simulink model "Controller_20231019"  (R2021b)
settings: Solver=ode4  StartTime=0.0  StopTime=5  FixedStep=0.01  RelTol=1e-3
values from neighbouring files (symbols this model uses):
  diag_M = diagonalize(M_frak0, M_frak)    [Initiate_KUKA_inv.m]
  iota0 = eye(6,6)    [Initiate_KUKA_inv.m]
  K_d = 10*[1.3*eye(3) zeros(3);zeros(3) 0.8*eye(3)]    [Initiate_FQ.m]    (also in Initiate_KUKA_inv.m = 5*[0.7*eye(3) zeros(3);zeros(3) 0.5*eye(3)])
  K_i = 5*[0.1*eye(3) zeros(3);zeros(3) 0.01*eye(3)]    [Initiate_FQ.m]    (also in Initiate_KUKA_inv.m = 5*[0.01*eye(3) zeros(3);zeros(3) 0.001*eye(3)])
  K_p = 100*[0.1 0 0 0 0 0;0 0.1 0 0 0 0; 0 0 0.1 0 0 0; 0 0 0 0.01 0 0 ... (first row only)    [Initiate_FQ.m]    (also in Initiate_KUKA_inv.m = 5*[0.1 0 0 0 0 0;0 0.1 0 0 0 0; 0 0 0.1 0 0 0; 0 0 0 0.01 0 )
  m0 = robot.Bodies{1,n+1}.Mass    [Initiate_KUKA_inv.m]
  M_t = (((Adjoint(g_It))'\M_t_body)/(Adjoint(g_It)))    [Initiate_FQ.m]    (also in Initiate_KUKA_inv.m = [eye(3)*mt zeros(3); zeros(3) eye(3)*80])
  mm = zeros(1,n)    [Initiate_KUKA_inv.m]
  mu = P0    [Initiate_FQ.m]    (also in Initiate_KUKA_inv.m = zeros(6,1))
  mu_t = inv((Adjoint(g_It))')*M_t_body*[V_It;w_t]    [Initiate_FQ.m]    (also in Initiate_KUKA_inv.m = M_t*[V_0t;w_t])
  q_dot_m = [0;0;0;0;0;0;0]    [Initiate_FQ.m]    (also in Initiate_KUKA_inv.m)
  q_m = [0.2;1.2;0.3;2.5;0.5;1.5;0.6]    [Initiate_FQ.m]    (also in Initiate_KUKA_inv.m = [0;0;0;0;0;0;0])
  rho_0t = [0.24;0.26;0.25]    [Initiate_KUKA_inv.m]
  sc_size = 1    [Initiate_KUKA_inv.m]
  V_0t = [-0.01;-0.01;0]    [Initiate_KUKA_inv.m]
  V_I0 = [-0.001;-0.001;0.0;-0.001;0.001;0.002]    [Initiate_FQ.m]    (also in Initiate_KUKA_inv.m = [0;0;0;0;0;0])
  Xi_m_matrix = zeros(6*n,n)    [Initiate_KUKA_inv.m]
undefined symbols (not defined in the file or in its folder): I0, Ie, Im, me, X, Xi_m, Y, Z
libraries: nesl_utility x83, sm_lib x78, robotcorelib x4
(part 4 of 4)

== system Controller_20231019/Space Manipulator1/joint//link5/iiwa_link_5 ==
  Inertia : sm_lib/Body Elements/Inertia  InertiaType=Custom  Mass=2.1633  MassUnits=kg  CenterOfMass=[0, 0, 0]  CenterOfMassUnits=m  MomentsOfInertia=[Im(1,1,5) Im(2,2,5) Im(3,3,5)]  MomentsOfInertiaUnits=kg*m^2  ProductsOfInertia=[Im(3,2,5) Im(3,1,5) Im(2,1,5)]  ProductsOfInertiaUnits=kg*m^2  GraphicType=None  MarkerShape=Inertia  MarkerSize=20  GraphicVisPropType=SimpleVisualProperties  GraphicDiffuseColor=[0.5 0.5 0.5]  GraphicSpecularColor=[0.5 0.5 0.5 1.0]  GraphicAmbientColor=[0.15 0.15 0.15 1.0]  GraphicEmissiveColor=[0.0 0.0 0.0 1.0]  GraphicShininess=75  GraphicOpacity=1.0
  ReferenceFrame : sm_lib/Frames and Transforms/Reference Frame
  Visual : sm_lib/Body Elements/File Solid  ExtGeomFileName=iiwa_description/meshes/iiwa7/visual/link_5.stl  UnitType=Custom  ExtGeomFileUnits=m  StepReaderType=HEX  ExportConvexHullGeometry=off  InertiaType=Custom  Mass=0  MassUnits=kg  CenterOfMass=[0, 0, 0]  CenterOfMassUnits=m  MomentsOfInertia=[0, 0, 0]  MomentsOfInertiaUnits=kg*m^2  ProductsOfInertia=[0, 0, 0]  ProductsOfInertiaUnits=kg*m^2  BasedOnType=DensityFromFile  Density=1000  DensityUnits=kg/m^3  DoExposeReferenceFrame=on  SerializedFrames=<Frames/>  GraphicType=FromGeometry  MarkerShape=Sphere  MarkerSize=10  GraphicVisPropType=SimpleVisualProperties  GraphicDiffuseColor=[1, 0.423529411765, 0.0392156862745]  GraphicSpecularColor=[0.5 0.5 0.5 1.0]  GraphicAmbientColor=[0.15 0.15 0.15 1.0]  GraphicEmissiveColor=[0.0 0.0 0.0 1.0]  GraphicShininess=75  GraphicOpacity=1
  VisualOriginTransform : sm_lib/Frames and Transforms/Rigid Transform  TranslationMethod=Cartesian  TranslationStandardOffset=0  TranslationLengthUnit=m  TranslationStandardAxis=+Z  TranslationCartesianOffset=[0, 0, -0.026]  TranslationROffset=0  TranslationROffsetUnits=m  TranslationZOffset=0  TranslationZOffsetUnits=m  TranslationThetaOffset=0  TranslationThetaOffsetUnits=deg  RotationMethod=RotationSequence  RotationAngleUnits=deg  RotationStandardAxis=+Z  RotationAngle=0.0  RotationArbitraryAxis=[0 0 1]  FollAlignAxisA=+X  BaseAlignAxisA=+Y  FollAlignAxisB=+Y  BaseAlignAxisB=+Z  RotationSequenceAxes=BaseAxes  RotationSequence=XYZ  RotationSequenceAngles=[0, 0, 0]  RotationSequenceAnglesUnits=rad  RotationMatrix=[1 0 0; 0 1 0; 0 0 1]
  iiwa_joint_5_AxisInvTransform : sm_lib/Frames and Transforms/Rigid Transform  TranslationMethod=Cartesian  TranslationStandardOffset=0  TranslationLengthUnit=m  TranslationStandardAxis=+Z  TranslationCartesianOffset=[0, 0, 0]  TranslationROffset=0  TranslationROffsetUnits=m  TranslationZOffset=0  TranslationZOffsetUnits=m  TranslationThetaOffset=0  TranslationThetaOffsetUnits=deg  RotationMethod=ArbitraryAxis  RotationAngleUnits=rad  RotationStandardAxis=+Z  RotationAngle=0  RotationArbitraryAxis=[1, 0, 0]  FollAlignAxisA=+X  BaseAlignAxisA=+Y  FollAlignAxisB=+Y  BaseAlignAxisB=+Z  RotationSequenceAxes=FollowerAxes  RotationSequence=XYX  RotationSequenceAngles=[0 0 0]  RotationSequenceAnglesUnits=deg  RotationMatrix=[1 0 0; 0 1 0; 0 0 1]
  iiwa_joint_6_AxisTransform : sm_lib/Frames and Transforms/Rigid Transform  TranslationMethod=Cartesian  TranslationStandardOffset=0  TranslationLengthUnit=m  TranslationStandardAxis=+Z  TranslationCartesianOffset=[0, 0, 0]  TranslationROffset=0  TranslationROffsetUnits=m  TranslationZOffset=0  TranslationZOffsetUnits=m  TranslationThetaOffset=0  TranslationThetaOffsetUnits=deg  RotationMethod=ArbitraryAxis  RotationAngleUnits=rad  RotationStandardAxis=+Z  RotationAngle=0  RotationArbitraryAxis=[1, 0, 0]  FollAlignAxisA=+X  BaseAlignAxisA=+Y  FollAlignAxisB=+Y  BaseAlignAxisB=+Z  RotationSequenceAxes=FollowerAxes  RotationSequence=XYX  RotationSequenceAngles=[0 0 0]  RotationSequenceAnglesUnits=deg  RotationMatrix=[1 0 0; 0 1 0; 0 0 1]
  iiwa_joint_6_OriginTransform : sm_lib/Frames and Transforms/Rigid Transform  TranslationMethod=Cartesian  TranslationStandardOffset=0  TranslationLengthUnit=m  TranslationStandardAxis=+Z  TranslationCartesianOffset=[0, 0.0607 , 0.19]  TranslationROffset=0  TranslationROffsetUnits=m  TranslationZOffset=0  TranslationZOffsetUnits=m  TranslationThetaOffset=0  TranslationThetaOffsetUnits=deg  RotationMethod=RotationSequence  RotationAngleUnits=deg  RotationStandardAxis=+Z  RotationAngle=0.0  RotationArbitraryAxis=[0 0 1]  FollAlignAxisA=+X  BaseAlignAxisA=+Y  FollAlignAxisB=+Y  BaseAlignAxisB=+Z  RotationSequenceAxes=BaseAxes  RotationSequence=XYZ  RotationSequenceAngles=[1.57079632679, 0, 0]  RotationSequenceAnglesUnits=rad  RotationMatrix=[1 0 0; 0 1 0; 0 0 1]
  F : PMIOPort  Side=Left
  F1 : PMIOPort  Port=2  Side=Right
  connections:
  iiwa_joint_5_AxisInvTransform/LConn1 -- iiwa_joint_6_OriginTransform/LConn1 -- Inertia/RConn1 -- ReferenceFrame/RConn1 -- VisualOriginTransform/LConn1
  Visual/RConn1 -- VisualOriginTransform/RConn1
  iiwa_joint_5_AxisInvTransform/RConn1 -- F/RConn1
  iiwa_joint_6_AxisTransform/RConn1 -- F1/RConn1
  iiwa_joint_6_AxisTransform/LConn1 -- iiwa_joint_6_OriginTransform/RConn1

== system Controller_20231019/Space Manipulator1/joint//link6/iiwa_link_6 ==
  Inertia : sm_lib/Body Elements/Inertia  InertiaType=Custom  Mass=2.3466  MassUnits=kg  CenterOfMass=[0, 0, 0]  CenterOfMassUnits=m  MomentsOfInertia=[Im(1,1,6) Im(2,2,6) Im(3,3,6)]  MomentsOfInertiaUnits=kg*m^2  ProductsOfInertia=[Im(3,2,6) Im(3,1,6) Im(2,1,6)]  ProductsOfInertiaUnits=kg*m^2  GraphicType=None  MarkerShape=Inertia  MarkerSize=20  GraphicVisPropType=SimpleVisualProperties  GraphicDiffuseColor=[0.5 0.5 0.5]  GraphicSpecularColor=[0.5 0.5 0.5 1.0]  GraphicAmbientColor=[0.15 0.15 0.15 1.0]  GraphicEmissiveColor=[0.0 0.0 0.0 1.0]  GraphicShininess=75  GraphicOpacity=1.0
  ReferenceFrame : sm_lib/Frames and Transforms/Reference Frame
  Visual : sm_lib/Body Elements/File Solid  ExtGeomFileName=iiwa_description/meshes/iiwa7/visual/link_6.stl  UnitType=Custom  ExtGeomFileUnits=m  StepReaderType=HEX  ExportConvexHullGeometry=off  InertiaType=Custom  Mass=0  MassUnits=kg  CenterOfMass=[0, 0, 0]  CenterOfMassUnits=m  MomentsOfInertia=[0, 0, 0]  MomentsOfInertiaUnits=kg*m^2  ProductsOfInertia=[0, 0, 0]  ProductsOfInertiaUnits=kg*m^2  BasedOnType=DensityFromFile  Density=1000  DensityUnits=kg/m^3  DoExposeReferenceFrame=on  SerializedFrames=<Frames/>  GraphicType=FromGeometry  MarkerShape=Sphere  MarkerSize=10  GraphicVisPropType=SimpleVisualProperties  GraphicDiffuseColor=[1, 0.423529411765, 0.0392156862745]  GraphicSpecularColor=[0.5 0.5 0.5 1.0]  GraphicAmbientColor=[0.15 0.15 0.15 1.0]  GraphicEmissiveColor=[0.0 0.0 0.0 1.0]  GraphicShininess=75  GraphicOpacity=1
  VisualOriginTransform : sm_lib/Frames and Transforms/Rigid Transform  TranslationMethod=Cartesian  TranslationStandardOffset=0  TranslationLengthUnit=m  TranslationStandardAxis=+Z  TranslationCartesianOffset=[0, 0, 0.0607 ]  TranslationROffset=0  TranslationROffsetUnits=m  TranslationZOffset=0  TranslationZOffsetUnits=m  TranslationThetaOffset=0  TranslationThetaOffsetUnits=deg  RotationMethod=RotationSequence  RotationAngleUnits=deg  RotationStandardAxis=+Z  RotationAngle=0.0  RotationArbitraryAxis=[0 0 1]  FollAlignAxisA=+X  BaseAlignAxisA=+Y  FollAlignAxisB=+Y  BaseAlignAxisB=+Z  RotationSequenceAxes=BaseAxes  RotationSequence=XYZ  RotationSequenceAngles=[0, 0, 0]  RotationSequenceAnglesUnits=rad  RotationMatrix=[1 0 0; 0 1 0; 0 0 1]
  iiwa_joint_6_AxisInvTransform : sm_lib/Frames and Transforms/Rigid Transform  TranslationMethod=Cartesian  TranslationStandardOffset=0  TranslationLengthUnit=m  TranslationStandardAxis=+Z  TranslationCartesianOffset=[0, 0, 0]  TranslationROffset=0  TranslationROffsetUnits=m  TranslationZOffset=0  TranslationZOffsetUnits=m  TranslationThetaOffset=0  TranslationThetaOffsetUnits=deg  RotationMethod=ArbitraryAxis  RotationAngleUnits=rad  RotationStandardAxis=+Z  RotationAngle=0  RotationArbitraryAxis=[1, 0, 0]  FollAlignAxisA=+X  BaseAlignAxisA=+Y  FollAlignAxisB=+Y  BaseAlignAxisB=+Z  RotationSequenceAxes=FollowerAxes  RotationSequence=XYX  RotationSequenceAngles=[0 0 0]  RotationSequenceAnglesUnits=deg  RotationMatrix=[1 0 0; 0 1 0; 0 0 1]
  iiwa_joint_7_AxisTransform : sm_lib/Frames and Transforms/Rigid Transform  TranslationMethod=Cartesian  TranslationStandardOffset=0  TranslationLengthUnit=m  TranslationStandardAxis=+Z  TranslationCartesianOffset=[0, 0, 0]  TranslationROffset=0  TranslationROffsetUnits=m  TranslationZOffset=0  TranslationZOffsetUnits=m  TranslationThetaOffset=0  TranslationThetaOffsetUnits=deg  RotationMethod=ArbitraryAxis  RotationAngleUnits=rad  RotationStandardAxis=+Z  RotationAngle=0  RotationArbitraryAxis=[1, 0, 0]  FollAlignAxisA=+X  BaseAlignAxisA=+Y  FollAlignAxisB=+Y  BaseAlignAxisB=+Z  RotationSequenceAxes=FollowerAxes  RotationSequence=XYX  RotationSequenceAngles=[0 0 0]  RotationSequenceAnglesUnits=deg  RotationMatrix=[1 0 0; 0 1 0; 0 0 1]
  iiwa_joint_7_OriginTransform : sm_lib/Frames and Transforms/Rigid Transform  TranslationMethod=Cartesian  TranslationStandardOffset=0  TranslationLengthUnit=m  TranslationStandardAxis=+Z  TranslationCartesianOffset=[0, 0.081, 0.0607 ]  TranslationROffset=0  TranslationROffsetUnits=m  TranslationZOffset=0  TranslationZOffsetUnits=m  TranslationThetaOffset=0  TranslationThetaOffsetUnits=deg  RotationMethod=RotationSequence  RotationAngleUnits=deg  RotationStandardAxis=+Z  RotationAngle=0.0  RotationArbitraryAxis=[0 0 1]  FollAlignAxisA=+X  BaseAlignAxisA=+Y  FollAlignAxisB=+Y  BaseAlignAxisB=+Z  RotationSequenceAxes=BaseAxes  RotationSequence=XYZ  RotationSequenceAngles=[-1.57079632679, 3.14159265359, 0]  RotationSequenceAnglesUnits=rad  RotationMatrix=[1 0 0; 0 1 0; 0 0 1]
  F : PMIOPort  Side=Left
  F1 : PMIOPort  Port=2  Side=Right
  connections:
  iiwa_joint_6_AxisInvTransform/LConn1 -- iiwa_joint_7_OriginTransform/LConn1 -- Inertia/RConn1 -- ReferenceFrame/RConn1 -- VisualOriginTransform/LConn1
  Visual/RConn1 -- VisualOriginTransform/RConn1
  iiwa_joint_6_AxisInvTransform/RConn1 -- F/RConn1
  iiwa_joint_7_AxisTransform/RConn1 -- F1/RConn1
  iiwa_joint_7_AxisTransform/LConn1 -- iiwa_joint_7_OriginTransform/RConn1

== system Controller_20231019/Space Manipulator1/joint//link7/iiwa_link_7 ==
  Inertia : sm_lib/Body Elements/Inertia  InertiaType=Custom  Mass=3.129  MassUnits=kg  CenterOfMass=[0, 0, 0]  CenterOfMassUnits=m  MomentsOfInertia=[Im(1,1,7) Im(2,2,7) Im(3,3,7)]  MomentsOfInertiaUnits=kg*m^2  ProductsOfInertia=[Im(3,2,7) Im(3,1,7) Im(2,1,7)]  ProductsOfInertiaUnits=kg*m^2  GraphicType=None  MarkerShape=Inertia  MarkerSize=20  GraphicVisPropType=SimpleVisualProperties  GraphicDiffuseColor=[0.5 0.5 0.5]  GraphicSpecularColor=[0.5 0.5 0.5 1.0]  GraphicAmbientColor=[0.15 0.15 0.15 1.0]  GraphicEmissiveColor=[0.0 0.0 0.0 1.0]  GraphicShininess=75  GraphicOpacity=1.0
  ReferenceFrame : sm_lib/Frames and Transforms/Reference Frame
  Visual : sm_lib/Body Elements/File Solid  ExtGeomFileName=iiwa_description/meshes/iiwa7/visual/link_7.stl  UnitType=Custom  ExtGeomFileUnits=m  StepReaderType=HEX  ExportConvexHullGeometry=off  InertiaType=Custom  Mass=0  MassUnits=kg  CenterOfMass=[0, 0, 0]  CenterOfMassUnits=m  MomentsOfInertia=[0, 0, 0]  MomentsOfInertiaUnits=kg*m^2  ProductsOfInertia=[0, 0, 0]  ProductsOfInertiaUnits=kg*m^2  BasedOnType=DensityFromFile  Density=1000  DensityUnits=kg/m^3  DoExposeReferenceFrame=on  SerializedFrames=<Frames/>  GraphicType=FromGeometry  MarkerShape=Sphere  MarkerSize=10  GraphicVisPropType=SimpleVisualProperties  GraphicDiffuseColor=[0.4, 0.4, 0.4]  GraphicSpecularColor=[0.5 0.5 0.5 1.0]  GraphicAmbientColor=[0.15 0.15 0.15 1.0]  GraphicEmissiveColor=[0.0 0.0 0.0 1.0]  GraphicShininess=75  GraphicOpacity=1
  VisualOriginTransform : sm_lib/Frames and Transforms/Rigid Transform  TranslationMethod=Cartesian  TranslationStandardOffset=0  TranslationLengthUnit=m  TranslationStandardAxis=+Z  TranslationCartesianOffset=[0, 0, -0.0005]  TranslationROffset=0  TranslationROffsetUnits=m  TranslationZOffset=0  TranslationZOffsetUnits=m  TranslationThetaOffset=0  TranslationThetaOffsetUnits=deg  RotationMethod=RotationSequence  RotationAngleUnits=deg  RotationStandardAxis=+Z  RotationAngle=0.0  RotationArbitraryAxis=[0 0 1]  FollAlignAxisA=+X  BaseAlignAxisA=+Y  FollAlignAxisB=+Y  BaseAlignAxisB=+Z  RotationSequenceAxes=BaseAxes  RotationSequence=XYZ  RotationSequenceAngles=[0, 0, 0]  RotationSequenceAnglesUnits=rad  RotationMatrix=[1 0 0; 0 1 0; 0 0 1]
  iiwa_joint_7_AxisInvTransform : sm_lib/Frames and Transforms/Rigid Transform  TranslationMethod=Cartesian  TranslationStandardOffset=0  TranslationLengthUnit=m  TranslationStandardAxis=+Z  TranslationCartesianOffset=[0, 0, 0]  TranslationROffset=0  TranslationROffsetUnits=m  TranslationZOffset=0  TranslationZOffsetUnits=m  TranslationThetaOffset=0  TranslationThetaOffsetUnits=deg  RotationMethod=ArbitraryAxis  RotationAngleUnits=rad  RotationStandardAxis=+Z  RotationAngle=0  RotationArbitraryAxis=[1, 0, 0]  FollAlignAxisA=+X  BaseAlignAxisA=+Y  FollAlignAxisB=+Y  BaseAlignAxisB=+Z  RotationSequenceAxes=FollowerAxes  RotationSequence=XYX  RotationSequenceAngles=[0 0 0]  RotationSequenceAnglesUnits=deg  RotationMatrix=[1 0 0; 0 1 0; 0 0 1]
  iiwa_joint_ee_OriginTransform : sm_lib/Frames and Transforms/Rigid Transform  TranslationMethod=Cartesian  TranslationStandardOffset=0  TranslationLengthUnit=m  TranslationStandardAxis=+Z  TranslationCartesianOffset=[0, 0, 0.045]  TranslationROffset=0  TranslationROffsetUnits=m  TranslationZOffset=0  TranslationZOffsetUnits=m  TranslationThetaOffset=0  TranslationThetaOffsetUnits=deg  RotationMethod=RotationSequence  RotationAngleUnits=deg  RotationStandardAxis=+Z  RotationAngle=0.0  RotationArbitraryAxis=[0 0 1]  FollAlignAxisA=+X  BaseAlignAxisA=+Y  FollAlignAxisB=+Y  BaseAlignAxisB=+Z  RotationSequenceAxes=BaseAxes  RotationSequence=XYZ  RotationSequenceAngles=[0, -1.57079632679, 0]  RotationSequenceAnglesUnits=rad  RotationMatrix=[1 0 0; 0 1 0; 0 0 1]
  iiwa_joint_ee_kuka_OriginTransform : sm_lib/Frames and Transforms/Rigid Transform  TranslationMethod=Cartesian  TranslationStandardOffset=0  TranslationLengthUnit=m  TranslationStandardAxis=+Z  TranslationCartesianOffset=[0, 0, 0.045]  TranslationROffset=0  TranslationROffsetUnits=m  TranslationZOffset=0  TranslationZOffsetUnits=m  TranslationThetaOffset=0  TranslationThetaOffsetUnits=deg  RotationMethod=RotationSequence  RotationAngleUnits=deg  RotationStandardAxis=+Z  RotationAngle=0.0  RotationArbitraryAxis=[0 0 1]  FollAlignAxisA=+X  BaseAlignAxisA=+Y  FollAlignAxisB=+Y  BaseAlignAxisB=+Z  RotationSequenceAxes=BaseAxes  RotationSequence=XYZ  RotationSequenceAngles=[3.14159265359, 3.14159265359, 3.14159265359]  RotationSequenceAnglesUnits=rad  RotationMatrix=[1 0 0; 0 1 0; 0 0 1]
  F : PMIOPort  Side=Left
  F2 : PMIOPort  Port=2  Side=Right
  F1 : PMIOPort  Port=3  Side=Right
  connections:
  Inertia/RConn1 -- ReferenceFrame/RConn1 -- iiwa_joint_ee_OriginTransform/LConn1 -- iiwa_joint_ee_kuka_OriginTransform/LConn1 -- iiwa_joint_7_AxisInvTransform/LConn1 -- VisualOriginTransform/LConn1
  Visual/RConn1 -- VisualOriginTransform/RConn1
  iiwa_joint_7_AxisInvTransform/RConn1 -- F/RConn1
  iiwa_joint_ee_OriginTransform/RConn1 -- F1/RConn1
  iiwa_joint_ee_kuka_OriginTransform/RConn1 -- F2/RConn1

== matlab function Controller_20231019/Dynamic Parameters/V_I0 ==
  data: P input; A_connection input; q_dot_m input; M0 input; V_I0 output
function V_I0=V_I0(P,A_connection,q_dot_m,M0)
% Find the spaccecraft velocity V_I0
% M0_inv=inv(M0);
% temp=P-transpose(A_connection)*q_dot_m;
V_I0=M0\P-A_connection*q_dot_m;

== matlab function Controller_20231019/Space Manipulator2/Q2q ==
  data: Q input; qm output
function qm = Q2q(Q)

qm=quat2eul(Q','XYZ')';

== matlab function Controller_20231019/Space Manipulator2/Q2q1 ==
  data: Q input; qm output
function qm = Q2q(Q)

qm=quat2eul(Q','XYZ')';

== matlab function Controller_20231019/Inverse Dynamics3/A_dot ==
  data: A_partial input; q_m input; A_dot output
function A_dot = fcn(A_partial, q_m)
n=length(q_m);

A_dot=zeros(6,n);
for i=1:n
    A_dot=A_dot+A_partial(:,:,i).*q_m(i);
end

== matlab function Controller_20231019/Inverse Dynamics3/C_hat/AMA_partial ==
  data: q_m input; AMA_partial output; M0 input; A input; A_partial input; V input; M0_partial input
function AMA_partial = AMA_partial(q_m,M0,A,A_partial,V,M0_partial)
% Calculates the C_hat_m matrix from base pose and arm joint angles

n=length(q_m);
b=length(V);

% find the temp intermediate term
AMA_partial=zeros(n,n,n);
for i=1:n
    AMA_partial(1:n,1:n,i)=transpose(A_partial(1:end,1:end,i))*M0*A+transpose(A)*M0_partial(1:end,1:end,i)*A+transpose(A)*M0*A_partial(1:end,1:end,i); %calcualte the derivative of not-augmented arm mass matrix from equation 121 of TRO paper
end

== matlab function Controller_20231019/Inverse Dynamics3/C_hat/A_partial ==
  data: q_m input; A_partial output; M0 input; M0_partial input; M0m_partial input; M0m input; V input
function A_partial = A_partial(q_m,M0,M0_partial,M0m_partial,M0m,V)
% Calculates the C_hat_m matrix from base pose and arm joint angles

n=length(q_m);
b=length(V);

% Find partial of connection A to each joint angle
A_partial=zeros(b,n,n);

temp1=zeros(b,n);
temp2=zeros(b,n);
temp3=zeros(b,n);

for i=1:n
    temp1=M0\(M0_partial(:,:,i));
    temp2=M0\M0m;
    temp3=M0\(M0m_partial(:,:,i));
    A_partial(1:b,1:n,i)=-temp1*temp2+temp3; % Equation 122
end

== matlab function Controller_20231019/Inverse Dynamics3/C_hat/C_hat1 ==
  data: q_m input; Mm_hat_partial input; q_dot_m input; C_hat output
function C_hat = C_hat(q_m, Mm_hat_partial,q_dot_m)
% Calculates the C_hat_m matrix from base pose and arm joint angles

n=length(q_m);


% Calculate C_hat matrix
C_temp1=zeros(n,n);
C_temp2=zeros(n,n);
C_hat=zeros(n,n);
for i=1:n
    C_temp1=C_temp1+squeeze(Mm_hat_partial(1:n,1:n,i)).*q_dot_m(i); % nxn by scalar
    C_temp2(i,1:n)=0.5*transpose(q_dot_m)*squeeze(Mm_hat_partial(1:n,1:n,i)); %1xn by nxn 
end

C_hat=C_temp1-C_temp2;

== matlab function Controller_20231019/Inverse Dynamics3/C_hat/Lm_partials/Lm0partial ==
  data: q_m input; Lm0_partial output; Xi_m input; iota0 input
function Lm0_partial = Lm0_partial(q_m,Xi_m,iota0)
% Calculates the C_hat_m matrix from base pose and arm joint angles

n=length(q_m);

% Find partial of Lm to joint angles
Lm0_partial=zeros(6*n,6,n); % 6nx6xn
for i=1:n
    for j=1:n
        Lm0_partial(6*(j-1)+1:6*j,1:6,i)=Ad_partial(j,1,i,Xi_m,q_m,iota0); % equation 114 of TRO paper
    end
end

%%%%%%%%%%%%%%%%%%%%%%%%%%%%%%%%%%%%%%%%%%%%%%%%%%%%%%%%%%%%% MUST BE
%%%%%%%%%%%%%%%%%%%%%%%%%%%%%%%%%%%%%%%%%%%%%%%%%%%%%%%%%%%%% CHECKED

== matlab function Controller_20231019/Inverse Dynamics3/C_hat/Lm_partials/Lmpartial ==
  data: q_m input; Lm_partial output; Xi_m input; iota0 input
function Lm_partial  = Lm_partial(q_m,Xi_m,iota0)
% Calculates the C_hat_m matrix from base pose and arm joint angles

n=length(q_m);

% Find partial of Lm0 to joint angles
Lm_partial=zeros(6*n,6*n,n); % 6nx6xn
for i=1:n
    Lm_partial(:,:,i)=zeros(6*n,6*n);
    for j=2:n
        for k=2:n
            if j>i && i>=k
                Lm_partial(6*(j-1)+1:6*j,6*(k-2)+1:6*(k-1),i)=Ad_partial(j,k,i,Xi_m,q_m,iota0); % equation 81 of TRO paper
            elseif i==j && i>=k
                Lm_partial(6*(j-1)+1:6*j,6*(k-2)+1:6*(k-1),i)=Ad_partial(j,k,i,Xi_m,q_m,iota0); % equation 81 of TRO paper
            else
                Lm_partial(6*(j-1)+1:6*(j-1)+6,6*(k-2)+1:6*(k-2)+6,i)=zeros(6,6);
            end

        end
    end
end

== matlab function Controller_20231019/Inverse Dynamics3/C_hat/M_partials/ M0partial ==
  data: q_m input; M0_partial output; Lm0 input; V input; iota0 input; diag_Mm input; Lm0_partial input
function M0_partial = M0_partial(q_m,Lm0,V,iota0,diag_Mm,Lm0_partial)
% Calculates the C_hat_m matrix from base pose and arm joint angles

n=length(q_m);
b=length(V);

% Find partial of M0 to joint angles
M0_partial=zeros(b,b,n); %initiate
for i=1:n
    temp1=transpose(Lm0_partial(1:end,1:end,i))*diag_Mm*Lm0;
    temp2=transpose(Lm0)*diag_Mm*Lm0_partial(1:end,1:end,i);
    M0_partial(1:b,1:b,i)= iota0'*(temp1+temp2)*iota0; %6x6 %equation 117 of TRO
end

== matlab function Controller_20231019/Inverse Dynamics3/C_hat/M_partials/M0mpartial ==
  data: q_m input; M0m_partial output; V input; Lm input; Lm0 input; iota0 input; diag_Mm input; Lm0_partial input; Lm_partial input; Xi_m_matrix input
function M0m_partial = M0m_partial(q_m,V,Lm,Lm0,iota0,diag_Mm,Lm0_partial,Lm_partial, Xi_m_matrix)
% Calculates the C_hat_m matrix from base pose and arm joint angles

n=length(q_m);
b=length(V);

% Find partial of M0m to joint angles
M0m_partial=zeros(b,n,n);
for i=1:n
    temp1=transpose(Lm0_partial(1:end,1:end,i))*diag_Mm*Lm;
    temp2=transpose(Lm0)*diag_Mm*Lm_partial(1:end,1:end,i);
    M0m_partial(1:b,1:n,i)= iota0'*(temp1+temp2)*Xi_m_matrix; % equation 118 of TRO paper
end

== matlab function Controller_20231019/Inverse Dynamics3/C_hat/M_partials/Mmpartial ==
  data: q_m input; Mm_partial output; Xi_m_matrix input; Lm input; diag_Mm input; Lm_partial input
function Mm_partial = Mm_partial(q_m,Xi_m_matrix,Lm,diag_Mm,Lm_partial)
% Calculates the C_hat_m matrix from base pose and arm joint angles

n=length(q_m);

% find the non-generalized arm mass matrix'x derivative to joint angles
Mm_partial=zeros(n,n,n);
for i=1:n
    temp=   transpose(Lm_partial(1:6*n,1:6*n,i))*diag_Mm*Lm  +   transpose(Lm)*diag_Mm*Lm_partial(1:6*n,1:6*n,i);
    Mm_partial(1:n,1:n,i)=transpose(Xi_m_matrix)*temp*Xi_m_matrix; %calcualte the derivative of not-augmented arm mass matrix from equation 120 of TRO paper
end

== matlab function Controller_20231019/Inverse Dynamics3/C_hat/Mm_hat_partial ==
  data: q_m input; AMA_partial input; Mm_hat_partial output; Mm_partial input
function Mm_hat_partial = Mm_hat_partial(q_m, AMA_partial, Mm_partial)
% Calculates the C_hat_m matrix from base pose and arm joint angles

n=length(q_m);

% find the generalized arm mass matrix'x derivative to joint angles
Mm_hat_partial=zeros(n,n,n);
for i=1:n
    Mm_hat_partial(1:n,1:n,i)=Mm_partial(1:n,1:n,i)-AMA_partial(1:n,1:n,i); %calcualte the derivative of augmented arm mass matrix from equation 119 of TRO paper
end

== matlab function Controller_20231019/Inverse Dynamics3/Inverse Dynamics/Ad_g_I0_dot ==
  data: g_I0 input; V_I0 input; Ad_g_I0_dot output
function Ad_g_I0_dot = Ad_g_I0_dot(g_I0,V_I0)
% Calculation of F_mu Eq 30 of paper
Ad_g_I0_dot=adjoint_low(V_I0)'*Adjoint(g_I0)';
% adjoint_low(V_I0)*transpose(Adjoint*(g_I0)))

== matlab function Controller_20231019/Inverse Dynamics3/Inverse Dynamics/Ad_g_I0_dot1 ==
  data: V_t input; Ad_g_It_dot output; g_It input
function Ad_g_It_dot = Ad_g_It_dot(V_t,g_It)
% Calculation of F_mu Eq 30 of paper
Ad_g_It_dot=adjoint_low(V_t)'*Adjoint(g_It)';

== matlab function Controller_20231019/Inverse Dynamics3/Inverse Dynamics/Ad_g_te_dot ==
  data: V_te input; Ad_g_te_dot output; g_te input
function Ad_g_te_dot = Ad_g_te_dot(V_te,g_te)
% Calculation of F_mu Eq 30 of paper
Ad_g_te_dot=-adjoint_low(V_te)/Adjoint(g_te);

== matlab function Controller_20231019/Inverse Dynamics3/Inverse Dynamics/FU ==
  data: MmJcross input; F_U output
function F_U = F_U(MmJcross)
F_U=MmJcross;

== matlab function Controller_20231019/Inverse Dynamics3/Inverse Dynamics/Fm ==
  data: MmJcross input; F_m output; A_dot input; Cm_hat input
function F_m = F_m(MmJcross,A_dot,Cm_hat)
% Calculation of F_mu Eq 30 of paper
F_m=MmJcross*(A_dot)+Cm_hat;

== matlab function Controller_20231019/										Controller/Velocity_error ==
  data: g_I0 input; V_Ie input; U_ff output; V_It input; V_It_dot input
function U_ff = U_ff(g_I0, V_Ie,V_It, V_It_dot)

U_ff=adjoint_low(V_Ie)*Adjoint(inv(g_I0))*V_It+Adjoint(inv(g_I0))*V_It_dot;

== matlab function Controller_20231019/Inverse Dynamics3/Inverse Dynamics/Fmu ==
  data: MmJcross input; M0 input; M_0_dot input; g_I0 input; F_mu output; Ad_g_I0_dot input
function F_mu = F_mu(MmJcross,M0,M_0_dot,g_I0,Ad_g_I0_dot)
% Calculation of F_mu Eq 30 of paper
F_mu=-MmJcross*(M0\M_0_dot*inv(M0)*transpose(Adjoint(g_I0))+ ...
    M0\Ad_g_I0_dot);

== matlab function Controller_20231019/Inverse Dynamics3/Inverse Dynamics/Inverse Dynamics ==
  data: F_mu output; F_t output; F_m output
function [F_mu,F_t,F_m] = fcn()


% n=length(q_m);

%Calculate Mass Matrix block components
% [ M0m Mm]=Mass_Matrix(q_m,Xi_m);

% A=inverse(M0)*M0m; % Mechanical Connection
% Mm_hat=Mm-transpose(A)*M0*A; %augmented manipulator mass matrix
% V=inverse(M0)*(mu-transpose(A)*q_dot_m); %Spacecraft Velocity

% The augmented Jacobian
% J_aug = J_em-J_e0*A;

% for i=1:n
%     for j=1:n
%         Cm_hat=
%     end
% end 

% Find A_dot thru finding partial of connection A to each joint angle
% A_partial=zeros(6,n,n);
% A_dot=zeros(6,n);
% for i=1:n
%     A_partial(6,n,i)=inverse(M0)*M0_partial(1:6,1:6,i)*inverse(M0)*M0m+inverse(M0)*M0m_partial(6,n,i); % Equation 122
%     A_dot(6,n)=A_dot+A_partial(6,n,i).*q_dot_m(i);
% end


% inverse or moore-penrose inverse of the augmented J2 Jacobian matrix
% if rank(J_aug)==size(J2(1,:))
%     J_inv=inverse(J2);
% else
%     J_inv=pinv(J2);
% end

% MJ_inv=-Mm_hat*J_cross;

% J_em_dot=J_em_dot;
% J_e0_dot=J_e0_dot;

% Form the eventual feedback transformation terms
% F_U=MmJcross; %done
% F_mu=MmJcross*(J_e0_dot*inverse(M0)*transpose(Adjoint*(g_I0))- ...
%     J_e0*inverse(M0)*M_0_dot*inverse(M0)*transpose(Adjoint*(g_I0))+ ...
%     J_e0*inverse(M0)*adjoint_low(inverse(M0*transpose(Adjoint(g_I0))*mu)-A*q_dot_m)); 
% F_t=MmJcross*();
% F_m=MmJcross*(J_em_dot-J_e0_dot*A-J_e0*A_dot)+Cm_hat;

== matlab function Controller_20231019/Inverse Dynamics3/Inverse Dynamics/MATLAB Function3 ==
  data: MmJcross input; g_te input; F_t output; g_It input; Mt input; Ad_gte_dot input; Ad_gIt_dot input
function F_t = F_t(MmJcross,g_te,g_It,Mt,Ad_gte_dot,Ad_gIt_dot)
% Calculation of F_mu Eq 30 of paper
F_t=-MmJcross*(Ad_gte_dot/Mt*Adjoint(g_It)'+Adjoint(g_te)\(Mt\Ad_gIt_dot));

% F_t=MmJcross*(-adjoint_low(V_te)/Adjoint(g_te)/Adjoint(g_tt)/M_t/Adjoint(g_It)'+...
%     Adjoint()\); 

% J_e0_dot*inverse(M0)*transpose(Adjoint*(g_I0))- ...
%     J_e0*inverse(M0)*M_0_dot*inverse(M0)*transpose(Adjoint*(g_I0))+ ...
%     J_e0*inverse(M0)*adjoint_low(inverse(M0*transpose(Adjoint(g_I0))*mu)-A*q_dot_m)
%     Ad_g_te_dot

== matlab function Controller_20231019/Inverse Dynamics3/Inverse Dynamics/MmJcross ==
  data: Mm_hat input; MmJcross output; A input
function MmJcross = MmJcross(Mm_hat, A)

JJ=-A;

% MmJcross = Mm_hat*pinv(JJ);
MmJcross = Mm_hat*pinv(JJ);

== matlab function Controller_20231019/Inverse Dynamics3/Inverse Dynamics/Mm_hat ==
  data: M0 input; Mm_hat output; Mm input; A input
function Mm_hat = Mm_hat(M0,Mm,A)

Mm_hat=Mm-A'*M0*A;

== matlab function Controller_20231019/Inverse Dynamics3/J augmented ==
  data: J_em input; J_aug output; J_e0 input; A input
function J_aug = fcn(J_em,J_e0,A)

== matlab function Controller_20231019/Inverse Dynamics3/M0_dot ==
  data: M0_partial input; q_m input; M0_dot output
function M0_dot = fcn(M0_partial, q_m)
n=length(q_m);

M0_dot=zeros(6,6);
for i=1:n
    M0_dot=M0_dot+M0_partial(:,:,i).*q_m(i);
end

== matlab function Controller_20231019/Inverse Dynamics3/MATLAB Function ==
  data: q_m input; q_dot_m input; Xi_m input; M0 input; M0m input; C_hat output; A input; V_I0 input
function C_hat = C_hat(q_m,q_dot_m,Xi_m,M0,M0m,A,V_I0)
% Calculates the C_hat_m matrix from base pose and arm joint angles

n=length(q_m);

% Find the connection A
% [M0, M0m, Mm]=Mass_Matrix(I0,Im,m0,mm,Tij,Ti0,q_m,Xi_m);
% A=inverse(M0)*M0m;

% Find the spaccecraft velocity V
% V=inverse(M0)*(P-transpose(A)*q_dot_m);
V=V_I0;

% Find Lm0
for i=1:n
    Lm0=Ad_frak(1,i,Xi_m,q_m);% equation 63 of TRO
end

% Find partial of Lm0 to joint angles
Lm0_partial=zeros(6*n,6,n); % 6nx6xn
for i=1:n
    for j=1:n
        Lm0_partial(6*(j-1)+1:6*j,1:6,i)=Ad_partial(j,1,i,Xi_m,q_m); % equation 114 of TRO paper
    end
end

% Find partial of M0 to joint angles
M0_partial=zeros(6,6,n); %initiate
for i=1:n
    M0_partial(1:6,1:6,i)= transpose(Lm0_partial(i))*diagM*Lm0+transpose(Lm0)*diagM*Lm0_partial(i); %6x6 %equation 117 of TRO
end

% Find partial of M0m to joint angles
M0m_partial=zeros(6,n,n);
for i=1:n
    M0m_partial(6,n,i)= (transpose(Lm0_partial)*diagM*Lm0+transpose(Lm0)*diagM*Lm)*Xi_m_matrix; % equation 118 of TRO paper
end

% Find partial of connection A to each joint angle
A_partial=zeros(6,n,n);
for i=1:n
    A_partial(6,n,i)=inverse(M0)*M0_partial(1:6,1:6,i)*inverse(M0)*M0m+inverse(M0)*M0m_partial(6,n,i); % Equation 122
end

% find the non-generalized arm mass matrix'x derivative to joint angles
for i=1:n
    Mm_partial(i)=transpose(Xi_m)*(transpose(Lm_partial(i))Lm + ...
        transpose(Lm)*()*Lm_partial(i))*Xi_m; %calcualte the derivative of not-augmented arm mass matrix from equation 120 of TRO paper
end

% find the temp intermediate term
for i=1:n
    AMA_partial(i)=transpose(A_partial(6,n,i))*M0*A+transpose(A)*M0_partial(i)*A+transpose(A)*M0*A_partial(6,n,i); %calcualte the derivative of not-augmented arm mass matrix from equation 121 of TRO paper
end

for i=1:n
    Mm_hat_partial(i)=Mm_partial(i)-AMA_partial(i); %calcualte the derivative of augmented arm mass matrix from equation 119 of TRO paper
end

for i=1:n
    C_temp1=C_temp1+Mm_hat_partial(n,n,i).*q_dot_m(i); % nxn by 1x1
    C_temp2()=0.5*transpose(q_dot_m)*Mm_hat_partial(n); %1xn by nx1 
end

C_hat=C_temp1-C_temp2;

== matlab function Controller_20231019/Inverse Dynamics3/MATLAB Function1 ==
  data: N_hat output; q_m input; q_dot_m input; Xi_m input; Xi_m_matrix input; M0 input; M0m input; A input; V_I0 input; P input
function N_hat = N_hat(q_m,q_dot_m,Xi_m,Xi_m_matrix, M0,M0m,A,V_I0,P)
% Calculates the N_hat_m matrix from base pose and arm joint angles

n=length(q_m);

V=V_I0;

% Find Lm0
for i=1:n
    Lm0=Ad_frak(1,i,Xi_m,q_m);% equation 63 of TRO
end

% Find partial of Lm0 to joint angles
Lm0_partial=zeros(6*n,6,n); % 6nx6xn
for i=1:n
    for j=1:n
        Lm0_partial(6*(j-1)+1:6*j,1:6,i)=Ad_partial(j,1,i,Xi_m,q_m); % equation 114 of TRO paper
    end
end

% Find partial of M0 to joint angles
M0_partial=zeros(6,6,n); %initiate
for i=1:n
    M0_partial(1:6,1:6,i)= transpose(Lm0_partial(i))*diagM*Lm0+transpose(Lm0)*diagM*Lm0_partial(i); %6x6 %equation 117 of TRO
end

% Find partial of M0m to joint angles
M0m_partial=zeros(6,n,n);
for i=1:n
    M0m_partial(6,n,i)= (transpose(Lm0_partial)*diagM*Lm0+transpose(Lm0)*diagM*Lm)*Xi_m_matrix; % equation 118 of TRO paper
end

% Find partial of connection A to each joint angle
A_partial=zeros(6,n,n);
for i=1:n
    A_partial(6,n,i)=inverse(M0)*M0_partial(1:6,1:6,i)*inverse(M0)*M0m+inverse(M0)*M0m_partial(6,n,i); % Equation 122
end


%Form N_hat from equation 19 of ACC paper
N_temp1=zeros(n,6); N_temp2=zeros(n,6); N_temp3=zeros(n,6);

for i=1:n
    N_temp1=N_temp1+transpose(A_partial(6,n,i).*q_dot_m(i)); % transpose of (6xn times 1x1)
    N_temp2(i,1:6)=transpose(q_dot_m)*transpose(A_partial(6,n,i)); %1xn times nx6
    N_temp3(i,1:6)=0.5*transpose(P)*M0_partial(1:6,1:6,i); % 1x6 times 6x6
end

N_hat=transpose(A)*transpose(adjoint_low(V))*P-N_temp1*P+N_temp2*P+N_temp3*P;

== matlab function Controller_20231019/Inverse Dynamics3/N_hat/N_hat ==
  data: N_hat_temp output; q_m input; q_dot_m input; A input; V input; P input; M0_partial input; A_partial input; iota0 input; M0 input
function N_hat_temp = N_hat(q_m,q_dot_m,A,V,P,M0_partial, A_partial, iota0, M0)
% Calculates the N_hat_m matrix from base pose and arm joint angles

n=length(q_m);
b=length(V);

%Form N_hat from equation 19 of ACC paper
N_temp1=zeros(n,b); N_temp2=zeros(n,b); N_temp3=zeros(n,b);

for i=1:n
    N_temp1=N_temp1+transpose(squeeze(A_partial(1:b,1:n,i)).*q_dot_m(i)); % transpose of (bxn times 1x1) 
    N_temp2(i,1:b)=transpose(q_dot_m)*transpose(squeeze(A_partial(1:b,1:n,i))); %1xn times nxb
    N_temp3(i,1:b)=0.5*transpose(P)*(-M0\M0_partial(1:end,1:end,i)/M0); % 1xb times bxb
end

N_hat_temp=transpose(A)*transpose(adjoint_low(V,iota0))-N_temp1+N_temp2+N_temp3;

== matlab function Controller_20231019/										Controller/gradient_of_Eg ==
  data: g_te input; Nabla_Eg output
function Nabla_Eg = fcn(g_te)

% Calculate the gradient of the Pose Error Function
p_te=g_te(1:3,4);
R_te=g_te(1:3,1:3);

temp=0.5*(R_te-transpose(R_te));

R_temp=vee3(temp);

Nabla_Eg=[p_te;R_temp];

== matlab function Controller_20231019/										Controller/Kinematics/g_te ==
  data: g_Ie input; g_It input; g_te output
function g_te = relative_pose(g_Ie, g_It)
% Calculates the relative pose of end-effector to target from the absolute
% poses of the end-effector and the target
g_te = inverse(g_It)*g_Ie;

== matlab function Controller_20231019/										Controller/Kinematics/Pose Error Function ==
  data: g_te input; E_g output
function E_g = pose_Error_function(g_te)
% Calculates the pose Error function from the relative pose of end-effector to target
R_te=g_te(1:3,1:3);
p_te=g_te(1:3,4);

temp_R=eye(3)-R_te;
temp_R=0.5*trace(temp_R);

temp_p=0.5*transpose(p_te)*p_te;
E_g =temp_R+temp_p;

== matlab function Controller_20231019/										Controller/Kinematics/Velocity_error ==
  data: g_I0 input; V_Ie input; V_e output; V_It input
function V_e = Velocity_Error_function(g_I0, V_Ie,V_It)
% Calculates the Velocity Error function from the momentums of chaser and
% target and the joint velocities

V_te_I=V_Ie-V_It;
V_te=Adjoint(inv(g_I0))*V_te_I;
V_e=V_te;

== matlab function Controller_20231019/Dynamic Parameters/MATLAB Function1 ==
  data: g_I0 input; mu input; P output
function P=Momentum(g_I0,mu)
% find the momentum in current base frame
P=transpose(Adjoint(g_I0))*mu;

== matlab function Controller_20231019/										Controller/Kinematics/velocity of target in EE ==
  data: g_te input; V_It_e output; V_It input
function V_It_e = V_It(g_te,V_It)
% Eq 25, second half
V_It_e=Adjoint(inv(g_te))*V_It;

== matlab function Controller_20231019/Dynamic Parameters/  ==
  data: q_m input; L0 output; Lm0 output; Lm output; Xi_m input
function [L0,Lm0,Lm] =L_calculator(q_m,Xi_m)
% Calculates the time-dependent L matrix
n=length(q_m);
L=zeros(6*(n+1),6*(n+1));
% Compute M_frak for ith body
% Calculate L matrix
for i=1:n+1
    for j=1:n+1
        if i>j
            Ad_temp=eye(6);
            for k=j:i-1
                Ad_temp=Adjoint(g_Matrix(-Xi_m(:,k),q_m(k)))*Ad_temp;
            end
            L(6*(i-1)+1:6*(i-1)+6,6*(j-1)+1:6*(j-1)+6)=Ad_temp;
        elseif i==j
            L(6*(i-1)+1:6*(i-1)+6,6*(j-1)+1:6*(j-1)+6)=eye(6);
        elseif i<j
            L(6*(i-1)+1:6*(i-1)+6,6*(j-1)+1:6*(j-1)+6)=zeros(6);
        end
    end
end

L0=L(1:6,1:6);
Lm0=L(7:end,1:6);
Lm=L(7:end,7:end);

end

== matlab function Controller_20231019/Dynamic Parameters/Mass Matrix Blocks/MATLAB Function ==
  data: diag_M input; m0_frak output; m_diag output
function [m0_frak,m_diag]=m_frak_decomp(diag_M)
% Compute the Mass Matrix of the multibody system.
%   Output:
%   M0      Spacecraft mass matrix 
%   M0m
%   Mm      Manipulator mass matrix

%n=length(q_m);

m0_frak=diag_M(1:6,1:6);
m_diag=diag_M(7:end,7:end);
